simulink model "Ex5_4_solution_simulink"  (R2019a)
settings: Solver=ode23tb  StartTime=0.0  StopTime=10.0  RelTol=1e-3
libraries: powerlib x10
settings Model: Creator=TomasJonsson  LastModifiedBy=TomasJonsson

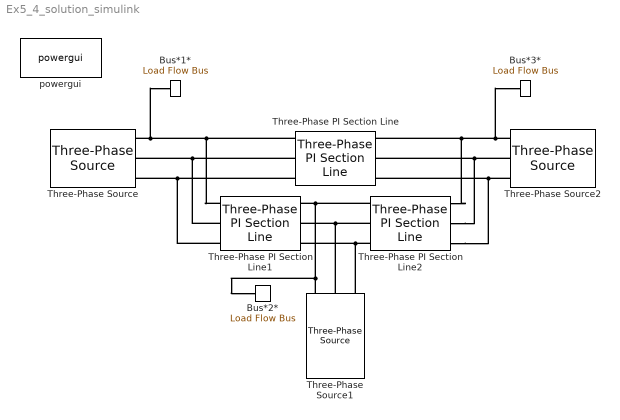
== system Ex5_4_solution_simulink ==
  Bus*1* : powerlib/Measurements/Load Flow Bus  LConnTagsString=a  Phases=single  Connectors=on one side  ID=Bus*1*  Vbase=345000  Vref=1  Vangle=0  VLF=1  VLFb=1  VLFc=1  angleLF=0  angleLFb=0  angleLFc=0
      settings: SourceProductName=Simscape Electrical
  Bus*2* : powerlib/Measurements/Load Flow Bus  LConnTagsString=a  Phases=single  Connectors=on one side  ID=Bus*2*  Vbase=345000  Vref=1.05  Vangle=0  VLF=1  VLFb=1  VLFc=1  angleLF=0  angleLFb=0  angleLFc=0
      settings: SourceProductName=Simscape Electrical
  Bus*3* : powerlib/Measurements/Load Flow Bus  LConnTagsString=a  Phases=single  Connectors=on one side  ID=Bus*3*  Vbase=345000  Vref=1  Vangle=0  VLF=1  VLFb=1  VLFc=1  angleLF=0  angleLFb=0  angleLFc=0
      settings: SourceProductName=Simscape Electrical
  Three-Phase PI Section Line : powerlib/Elements/Three-Phase PI Section Line  LConnTagsString=a|b|c  RConnTagsString=A|B|C  Frequency=60  Resistances=[ 0.037 0.037]  Inductances="[ 1e-3  1e-3]"  Capacitances=[11.9e-9 11.9e-9]  Length=200
      settings: SourceProductName=Simscape Electrical
  Three-Phase PI Section Line1 : powerlib/Elements/Three-Phase PI Section Line  LConnTagsString=a|b|c  RConnTagsString=A|B|C  Frequency=60  Resistances=[ 0.037 0.037]  Inductances="[ 1e-3  1e-3]"  Capacitances=[11.9e-9 11.9e-9]  Length=150
      settings: SourceProductName=Simscape Electrical
  Three-Phase PI Section Line2 : powerlib/Elements/Three-Phase PI Section Line  LConnTagsString=a|b|c  RConnTagsString=A|B|C  Frequency=60  Resistances=[ 0.037 0.037]  Inductances="[ 1e-3  1e-3]"  Capacitances=[11.9e-9 11.9e-9]  Length=150
      settings: SourceProductName=Simscape Electrical
  Three-Phase Source : powerlib/Electrical Sources/Three-Phase Source  InternalConnection=Yg  VoltagePhases=off  Voltage=345e3  PhaseAngle=0  Voltage_phases=[25e3 25e3 25e3]/sqrt(3)  PhaseAngles_phases=[0 -120 +120]  Frequency=60  NonIdealSource=on  SpecifyImpedance=off  Resistance=0.01  Inductance=0  ShortCircuitLevel=100e6  BaseVoltage=345e3  XRratio=7  BusType=swing  Pref=10e3  Qref=0  Prefabc=[10e3, 10e3, 10e3]  Qrefabc=[0, 0, 0]  Qmin=-inf  Qmax=inf
      settings: SourceProductName=Simscape Electrical
  Three-Phase Source1 : powerlib/Electrical Sources/Three-Phase Source  InternalConnection=Yg  VoltagePhases=off  Voltage=345e3  PhaseAngle=0  Voltage_phases=[25e3 25e3 25e3]/sqrt(3)  PhaseAngles_phases=[0 -120 +120]  Frequency=60  NonIdealSource=on  SpecifyImpedance=off  Resistance=0.01  Inductance=0  ShortCircuitLevel=100e6  BaseVoltage=345e3  XRratio=7  BusType=PV  Pref=200e6  Qref=0  Prefabc=[10e3, 10e3, 10e3]  Qrefabc=[0, 0, 0]  Qmin=-inf  Qmax=inf
      settings: SourceProductName=Simscape Electrical
  Three-Phase Source2 : powerlib/Electrical Sources/Three-Phase Source  InternalConnection=Yg  VoltagePhases=off  Voltage=345e3  PhaseAngle=0  Voltage_phases=[25e3 25e3 25e3]/sqrt(3)  PhaseAngles_phases=[0 -120 +120]  Frequency=60  NonIdealSource=on  SpecifyImpedance=off  Resistance=0.01  Inductance=0  ShortCircuitLevel=100e6  BaseVoltage=345e3  XRratio=7  BusType=PQ  Pref=-500e6  Qref=-100e6  Prefabc=[10e3, 10e3, 10e3]  Qrefabc=[0, 0, 0]  Qmin=-inf  Qmax=inf
      settings: SourceProductName=Simscape Electrical
  powergui : powerlib/powergui  Priority=1  SimulationMode=Phasor  SampleTime=50e-6  frequency=60  Iterations=50  frequencyindice=60  Pbase=100e6  ErrMax=1e-4  UnitsV=kV  UnitsW=MW  buscounter=3  FunctionMessages=off  echomessages=off  EnableUseOfTLC=off  CurrentSourceSwitches=off  DisableSnubberDevices=off  DisableRonSwitches=off  DisableVfSwitches=off  DisplayEquations=off  AutomaticDiscreteSolvers=off  SolverType=Tustin/Backward Euler (TBE)  Interpol=off  ExternalGateDelay=off  methode=off  Ts=100  x0status=blocks  SPID=on  SwTol=0  HookPort=off  NonlinearTolerance=0  nMaxIteration=15  ContinueOnMaxIteration=off  RestoreLinks=warning  ResistiveCurrentMeasurement=off  Frange=[0:2:500]  Ylog=off  Xlog=on  ShowGrid=off  save=off  variable=ZData  structure=0  ZoomFFT=off  StartTime=0.0  cycles=1  DisplayStyle=1  fundamental=60  FreqAxis=off  MaxFrequency=1000  frequencyindicesteady=1  RmsSteady=1  display=off
      settings: SourceProductName=Simscape Electrical
  connections:
  Three-Phase PI Section Line/LConn1 -- Three-Phase PI Section Line1/LConn1 -- Three-Phase Source/RConn1 -- Bus*1*/LConn1
  Three-Phase PI Section Line/LConn2 -- Three-Phase PI Section Line1/LConn2 -- Three-Phase Source/RConn2
  Three-Phase PI Section Line/LConn3 -- Three-Phase PI Section Line1/LConn3 -- Three-Phase Source/RConn3
  Three-Phase Source2/RConn1 -- Bus*3*/LConn1 -- Three-Phase PI Section Line2/RConn1 -- Three-Phase PI Section Line/RConn1
  Three-Phase Source2/RConn2 -- Three-Phase PI Section Line2/RConn2 -- Three-Phase PI Section Line/RConn2
  Three-Phase Source2/RConn3 -- Three-Phase PI Section Line2/RConn3 -- Three-Phase PI Section Line/RConn3
  Three-Phase PI Section Line2/LConn1 -- Three-Phase Source1/RConn1 -- Bus*2*/LConn1 -- Three-Phase PI Section Line1/RConn1
  Three-Phase PI Section Line2/LConn2 -- Three-Phase Source1/RConn2 -- Three-Phase PI Section Line1/RConn2
  Three-Phase PI Section Line2/LConn3 -- Three-Phase PI Section Line1/RConn3 -- Three-Phase Source1/RConn3
